simulink library "DEM_lib"  (Simulink 7.4)
settings: Solver=FixedStepDiscrete  StartTime=0.0  StopTime=Inf  FixedStep=0.001  RelTol=1e-3
undefined symbols (not defined in the file or in its folder): BCU_Drive_St, BCU_FastCharge_St, BCU_SlowCharge_St, COR_Fault_Bus, CTC_DefaultOffline_CtrCmd, CTC_DriveEmgyDcnct_CtrCmd, CTC_DriveOffline_CtrCmd, CTC_DriveOnline_CtrCmd, EHP_Fault_Bus, FCM_Fault_Bus, SCM_Fault_Bus
libraries: Defined_Functionality x82, simulink x2
(part 4 of 4)

== system DEM_lib/Diagnostic_Event_Management/Level_handle/DRIVE/FaultLevelConfirmed/LvlErr1 ==
  Err : Inport
  Bus Selector : BusSelector  OutputSignals=BPN_Fault_Bus.BPNd_cflt_CellVoltOver_warnRaw,BPN_Fault_Bus.BPNd_cflt_CellVoltUnder_warnRaw,BPN_Fault_Bus.BPNd_cflt_CellVoltDifOver_warnRaw,BPN_Fault_Bus.BPNd_cflt_PackVoltOver_warnRaw,BPN_Fault_Bus.BPNd_cflt_PackVoltUnder_warnRaw,BPN_Fault_Bus.BPNd_cflt_ChaCurOver_warnRaw,BPN_Fault_Bus.BPNd_cflt_DchCurOver_warnRaw,BPN_Fault_Bus.BPNd_cflt_PackSocUnder_warnRaw,BPN_Fault_Bus.BPNd_cflt_PackSocOver_warnRaw,BPN_Fault_Bus.BPNd_cflt_PulChaPowOver_warnRaw,BPN_Fault_Bus.BPNd_cflt_PulDchPowOver_warnRaw,BAL_Fault_Bus.BALd_cflt_BalSwthAnml_warnRaw,BTM_Fault_Bus.BTMd_cflt_MdlTempOver_warnRaw,BTM_Fault_Bus.BTMd_cflt_BMUMaxTempOver_warnRaw,BTM_Fault_Bus.BTMd_cflt_BCUMaxTempOver_warnRaw,BTM_Fault_Bus.BTMd_cflt_MdlTempUnder_warnRaw,BTM_Fault_Bus.BTMd_cflt_MdlTempDifOver_warnRaw,IPT_Fault_Bus.IPTd_cflt_CC2CnctSt_warnRaw,IPT_Fault_Bus.IPTd_cflt_CCCnctSt_warnRaw,IPT_Fault_Bus.IPTd_cflt_VMSCANMsg_faultRaw,IPT_Fault_Bus.IPTd_cflt_KL30Raw,IPT_Fault_Bus.IPTd_cflt_MSDVoltRaw,IPT_Fault_Bus.IPTd_cflt_PCBTempRaw,IPT_Fault_Bus.IPTd_cflt_PosCtrVoltRef1_backRaw,IPT_Fault_Bus.IPTd_cflt_PosCtrVoltRef1_frontRaw,IPT_Fault_Bus.IPTd_cflt_PosCtrVoltRef2_backRaw,IPT_Fault_Bus.IPTd_cflt_PosCtrVoltRef2_frontRaw,IPT_Fault_Bus.IPTd_cflt_ShuntCurRaw,IPT_Fault_Bus.IPTd_cflt_USampleRaw
  Constant : Constant  OutDataTypeMode=uint8  OutDataTypeStr=uint8
  Constant1 : Constant  Value=0  OutDataTypeMode=uint8  OutDataTypeStr=uint8
  Logical Operator : Logic  Operator=OR  Inputs=29  AllPortsSameDT=off  OutDataTypeMode=boolean  OutDataTypeStr=boolean
  Switch : Switch  Criteria=u2 ~= 0
  ErrLvl : Outport
  wires:
  Bus Selector/29 -> Logical Operator/29  "<IPTd_cflt_USampleRaw>"
  Bus Selector/28 -> Logical Operator/28  "<IPTd_cflt_ShuntCurRaw>"
  Bus Selector/27 -> Logical Operator/27  "<IPTd_cflt_PosCtrVoltRef2_frontRaw>"
  Bus Selector/26 -> Logical Operator/26  "<IPTd_cflt_PosCtrVoltRef2_backRaw>"
  Bus Selector/25 -> Logical Operator/25  "<IPTd_cflt_PosCtrVoltRef1_frontRaw>"
  Bus Selector/24 -> Logical Operator/24  "<IPTd_cflt_PosCtrVoltRef1_backRaw>"
  Bus Selector/23 -> Logical Operator/23  "<IPTd_cflt_PCBTempRaw>"
  Bus Selector/22 -> Logical Operator/22  "<IPTd_cflt_MSDVoltRaw>"
  Bus Selector/21 -> Logical Operator/21  "<IPTd_cflt_KL30Raw>"
  Bus Selector/20 -> Logical Operator/20  "<IPTd_cflt_VMSCANMsg_faultRaw>"
  Bus Selector/19 -> Logical Operator/19  "<IPTd_cflt_CCCnctSt_warnRaw>"
  Bus Selector/18 -> Logical Operator/18  "<IPTd_cflt_CC2CnctSt_warnRaw>"
  Bus Selector/17 -> Logical Operator/17  "<BTMd_cflt_MdlTempDifOver_warnRaw>"
  Bus Selector/16 -> Logical Operator/16  "<BTMd_cflt_MdlTempUnder_warnRaw>"
  Bus Selector/15 -> Logical Operator/15  "<BTMd_cflt_BCUMaxTempOver_warnRaw>"
  Bus Selector/14 -> Logical Operator/14  "<BTMd_cflt_BMUMaxTempOver_warnRaw>"
  Bus Selector/13 -> Logical Operator/13  "<BTMd_cflt_MdlTempOver_warnRaw>"
  Bus Selector/12 -> Logical Operator/12  "<BALd_cflt_BalSwthAnml_warnRaw>"
  Bus Selector/11 -> Logical Operator/11  "<BPNd_cflt_PulDchPowOver_warnRaw>"
  Bus Selector/10 -> Logical Operator/10  "<BPNd_cflt_PulChaPowOver_warnRaw>"
  Bus Selector/9 -> Logical Operator/9  "<BPNd_cflt_PackSocOver_warnRaw>"
  Bus Selector/8 -> Logical Operator/8  "<BPNd_cflt_PackSocUnder_warnRaw>"
  Bus Selector/7 -> Logical Operator/7  "<BPNd_cflt_DchCurOver_warnRaw>"
  Bus Selector/6 -> Logical Operator/6  "<BPNd_cflt_ChaCurOver_warnRaw>"
  Bus Selector/5 -> Logical Operator/5  "<BPNd_cflt_PackVoltUnder_warnRaw>"
  Bus Selector/4 -> Logical Operator/4  "<BPNd_cflt_PackVoltOver_warnRaw>"
  Bus Selector/3 -> Logical Operator/3  "<BPNd_cflt_CellVoltDifOver_warnRaw>"
  Bus Selector/2 -> Logical Operator/2  "<BPNd_cflt_CellVoltUnder_warnRaw>"
  Switch/1 -> ErrLvl/1
  Constant1/1 -> Switch/3
  Constant/1 -> Switch/1
  Logical Operator/1 -> Switch/2
  Err/1 -> Bus Selector/1
  Bus Selector/1 -> Logical Operator/1  "<BPNd_cflt_CellVoltOver_warnRaw>"

== system DEM_lib/Diagnostic_Event_Management/Level_handle/DRIVE/FaultLevelConfirmed/LvlErr2 ==
  Err : Inport
  Bus Selector : BusSelector  OutputSignals=BPN_Fault_Bus.BPNd_cflt_CellVoltOver_faultRaw,BPN_Fault_Bus.BPNd_cflt_CellVoltUnder_faultRaw,BPN_Fault_Bus.BPNd_cflt_CellVoltDifOver_faultRaw,BPN_Fault_Bus.BPNd_cflt_PackVoltOver_faultRaw,BPN_Fault_Bus.BPNd_cflt_PackVoltUnder_faultRaw,BPN_Fault_Bus.BPNd_cflt_ChaCurOver_faultRaw,BPN_Fault_Bus.BPNd_cflt_DchCurOver_faultRaw,BPN_Fault_Bus.BPNd_cflt_PackSocUnder_faultRaw,BPN_Fault_Bus.BPNd_cflt_PackSocOver_faultRaw,BPN_Fault_Bus.BPNd_cflt_PulChaPowOver_faultRaw,BPN_Fault_Bus.BPNd_cflt_PulDchPowOver_faultRaw,BPN_Fault_Bus.BPNd_cflt_PackInRes_fatalRaw,BPN_Fault_Bus.BPNd_cflt_HVPosCtrlR_faultRaw,BPN_Fault_Bus.BPNd_cflt_HVNegCtrlR_faultRaw,BPN_Fault_Bus.BPNd_cflt_HVAcq_warnRaw,EHP_Fault_Bus.EHPd_cflt_NegIso_warnRaw,EHP_Fault_Bus.EHPd_cflt_PosIso_warnRaw,COR_Fault_Bus.CORd_cflt_CellCDcse_faultRaw,COR_Fault_Bus.CORd_cflt_CellRDcse_faultRaw,COR_Fault_Bus.CORd_cflt_CellRIcse_faultRaw,BTM_Fault_Bus.BTMd_cflt_MdlTempOver_faultRaw,BTM_Fault_Bus.BTMd_cflt_MdlTempDifOver_faultRaw
  Constant : Constant  Value=2  OutDataTypeMode=uint8  OutDataTypeStr=uint8
  Constant1 : Constant  Value=0  OutDataTypeMode=uint8  OutDataTypeStr=uint8
  Logical Operator : Logic  Operator=OR  Inputs=22  AllPortsSameDT=off  OutDataTypeMode=boolean  OutDataTypeStr=boolean
  Switch : Switch  Criteria=u2 ~= 0
  ErrLvl : Outport
  wires:
  Bus Selector/22 -> Logical Operator/22  "<BTMd_cflt_MdlTempDifOver_faultRaw>"
  Bus Selector/21 -> Logical Operator/21  "<BTMd_cflt_MdlTempOver_faultRaw>"
  Bus Selector/20 -> Logical Operator/20  "<CORd_cflt_CellRIcse_faultRaw>"
  Bus Selector/19 -> Logical Operator/19  "<CORd_cflt_CellRDcse_faultRaw>"
  Bus Selector/18 -> Logical Operator/18  "<CORd_cflt_CellCDcse_faultRaw>"
  Bus Selector/17 -> Logical Operator/17  "<EHPd_cflt_PosIso_warnRaw>"
  Bus Selector/16 -> Logical Operator/16  "<EHPd_cflt_NegIso_warnRaw>"
  Bus Selector/15 -> Logical Operator/15  "<BPNd_cflt_HVAcq_warnRaw>"
  Bus Selector/14 -> Logical Operator/14  "<BPNd_cflt_HVNegCtrlR_faultRaw>"
  Bus Selector/13 -> Logical Operator/13  "<BPNd_cflt_HVPosCtrlR_faultRaw>"
  Bus Selector/12 -> Logical Operator/12  "<BPNd_cflt_PackInRes_fatalRaw>"
  Bus Selector/11 -> Logical Operator/11  "<BPNd_cflt_PulDchPowOver_faultRaw>"
  Bus Selector/10 -> Logical Operator/10  "<BPNd_cflt_PulChaPowOver_faultRaw>"
  Bus Selector/9 -> Logical Operator/9  "<BPNd_cflt_PackSocOver_faultRaw>"
  Bus Selector/8 -> Logical Operator/8  "<BPNd_cflt_PackSocUnder_faultRaw>"
  Bus Selector/7 -> Logical Operator/7  "<BPNd_cflt_DchCurOver_faultRaw>"
  Bus Selector/6 -> Logical Operator/6  "<BPNd_cflt_ChaCurOver_faultRaw>"
  Bus Selector/5 -> Logical Operator/5  "<BPNd_cflt_PackVoltUnder_faultRaw>"
  Bus Selector/4 -> Logical Operator/4  "<BPNd_cflt_PackVoltOver_faultRaw>"
  Bus Selector/3 -> Logical Operator/3  "<BPNd_cflt_CellVoltDifOver_faultRaw>"
  Bus Selector/2 -> Logical Operator/2  "<BPNd_cflt_CellVoltUnder_faultRaw>"
  Switch/1 -> ErrLvl/1
  Constant1/1 -> Switch/3
  Constant/1 -> Switch/1
  Bus Selector/1 -> Logical Operator/1  "<BPNd_cflt_CellVoltOver_faultRaw>"
  Err/1 -> Bus Selector/1
  Logical Operator/1 -> Switch/2

== system DEM_lib/Diagnostic_Event_Management/Level_handle/DRIVE/FaultLevelConfirmed/LvlErr3 ==
  Err : Inport
  Bus Selector : BusSelector  OutputSignals=BPN_Fault_Bus.BPNd_cflt_CellVoltOver_fatalRaw,BPN_Fault_Bus.BPNd_cflt_CellVoltUnder_fatalRaw,BPN_Fault_Bus.BPNd_cflt_PackVoltOver_fatalRaw,BPN_Fault_Bus.BPNd_cflt_PackVoltUnder_fatalRaw,BPN_Fault_Bus.BPNd_cflt_ChaCurOver_fatalRaw,BPN_Fault_Bus.BPNd_cflt_DchCurOver_fatalRaw,BPN_Fault_Bus.BPNd_cflt_PulChaPowOver_fatalRaw,BPN_Fault_Bus.BPNd_cflt_PulDchPowOver_fatalRaw,BPN_Fault_Bus.BPNd_cflt_PackVoltDrop_fatalRaw,CTC_Fault_Bus.CTCd_cflt_PosCtrStuckOpen_faultRaw,CTC_Fault_Bus.CTCd_cflt_PosCtrStuckCld_faultRaw,CTC_Fault_Bus.CTCd_cflt_NegCtrStuckOpen_faultRaw,CTC_Fault_Bus.CTCd_cflt_NegCtrStuckCld_faultRaw,CTC_Fault_Bus.CTCd_cflt_PrecTmOver_faultRaw,CTC_Fault_Bus.CTCd_cflt_HVCnctTmOver_faultRaw,CTC_Fault_Bus.CTCd_cflt_HVDcncWaitTmOver_faultRaw,CTC_Fault_Bus.CTCd_cflt_HVDcnctTmOver_faultRaw,CTC_Fault_Bus.CTCd_cflt_HVEmcyDcnctTmOver_faultRaw,CTC_Fault_Bus.CTCd_cflt_PrecCurOver_faultRaw,CTC_Fault_Bus.CTCd_cflt_HVCnctCurOver_faultRaw,EHP_Fault_Bus.EHPd_cflt_NegIso_faultRaw,EHP_Fault_Bus.EHPd_cflt_PosIso_faultRaw,EHP_Fault_Bus.EHPd_cflt_HVILSt_faultRaw,BTM_Fault_Bus.BTMd_cflt_MdlTempOver_fatalRaw,BSC_Fault_Bus.BSCd_cflt_BCUFaultRaw,MCC_Fault_Bus.MCCd_cflt_BMUInit_faultRaw
  Constant : Constant  Value=3  OutDataTypeMode=uint8  OutDataTypeStr=uint8
  Constant1 : Constant  Value=0  OutDataTypeMode=uint8  OutDataTypeStr=uint8
  Logical Operator1 : Logic  Operator=OR  Inputs=26  AllPortsSameDT=off  OutDataTypeMode=boolean  OutDataTypeStr=boolean
  Switch : Switch  Criteria=u2 ~= 0
  ErrLvl : Outport
  wires:
  Bus Selector/26 -> Logical Operator1/26  "<MCCd_cflt_BMUInit_faultRaw>"
  Bus Selector/25 -> Logical Operator1/25  "<BSCd_cflt_BCUFaultRaw>"
  Bus Selector/24 -> Logical Operator1/24  "<BTMd_cflt_MdlTempOver_fatalRaw>"
  Bus Selector/23 -> Logical Operator1/23  "<EHPd_cflt_HVILSt_faultRaw>"
  Bus Selector/22 -> Logical Operator1/22  "<EHPd_cflt_PosIso_faultRaw>"
  Bus Selector/21 -> Logical Operator1/21  "<EHPd_cflt_NegIso_faultRaw>"
  Bus Selector/20 -> Logical Operator1/20  "<CTCd_cflt_HVCnctCurOver_faultRaw>"
  Bus Selector/19 -> Logical Operator1/19  "<CTCd_cflt_PrecCurOver_faultRaw>"
  Bus Selector/18 -> Logical Operator1/18  "<CTCd_cflt_HVEmcyDcnctTmOver_faultRaw>"
  Bus Selector/17 -> Logical Operator1/17  "<CTCd_cflt_HVDcnctTmOver_faultRaw>"
  Bus Selector/16 -> Logical Operator1/16  "<CTCd_cflt_HVDcncWaitTmOver_faultRaw>"
  Bus Selector/15 -> Logical Operator1/15  "<CTCd_cflt_HVCnctTmOver_faultRaw>"
  Bus Selector/14 -> Logical Operator1/14  "<CTCd_cflt_PrecTmOver_faultRaw>"
  Bus Selector/13 -> Logical Operator1/13  "<CTCd_cflt_NegCtrStuckCld_faultRaw>"
  Bus Selector/12 -> Logical Operator1/12  "<CTCd_cflt_NegCtrStuckOpen_faultRaw>"
  Bus Selector/11 -> Logical Operator1/11  "<CTCd_cflt_PosCtrStuckCld_faultRaw>"
  Bus Selector/10 -> Logical Operator1/10  "<CTCd_cflt_PosCtrStuckOpen_faultRaw>"
  Bus Selector/9 -> Logical Operator1/9  "<BPNd_cflt_PackVoltDrop_fatalRaw>"
  Bus Selector/8 -> Logical Operator1/8  "<BPNd_cflt_PulDchPowOver_fatalRaw>"
  Bus Selector/7 -> Logical Operator1/7  "<BPNd_cflt_PulChaPowOver_fatalRaw>"
  Bus Selector/6 -> Logical Operator1/6  "<BPNd_cflt_DchCurOver_fatalRaw>"
  Bus Selector/5 -> Logical Operator1/5  "<BPNd_cflt_ChaCurOver_fatalRaw>"
  Bus Selector/4 -> Logical Operator1/4  "<BPNd_cflt_PackVoltUnder_fatalRaw>"
  Bus Selector/3 -> Logical Operator1/3  "<BPNd_cflt_PackVoltOver_fatalRaw>"
  Bus Selector/2 -> Logical Operator1/2  "<BPNd_cflt_CellVoltUnder_fatalRaw>"
  Switch/1 -> ErrLvl/1
  Constant1/1 -> Switch/3
  Constant/1 -> Switch/1
  Logical Operator1/1 -> Switch/2
  Err/1 -> Bus Selector/1
  Bus Selector/1 -> Logical Operator1/1  "<BPNd_cflt_CellVoltOver_fatalRaw>"

== system DEM_lib/Diagnostic_Event_Management/Level_handle/DRIVE/handle/DriveCtrCmdRaw ==
  BSCd_enum_BCUSt : Inport
  IPTd_flg_VehHVCnctCmd : Inport  Port=2
  Compare To Constant4 : simulink/Logic and Bit Operations/Compare To Constant  SystemSampleTime=-1  relop===  const=BCU_Drive_St  LogicOutDataTypeMode=uint8
  Compare To Constant5 : simulink/Logic and Bit Operations/Compare To Constant  SystemSampleTime=-1  relop===  const=1  LogicOutDataTypeMode=uint8
  Constant1 : Constant  Value=CTC_DriveOffline_CtrCmd  OutDataTypeMode=uint8  OutDataTypeStr=uint8
  Constant2 : Constant  Value=CTC_DriveOnline_CtrCmd  OutDataTypeMode=uint8  OutDataTypeStr=uint8
  Logical Operator3 : Logic  AllPortsSameDT=off  OutDataTypeMode=boolean  OutDataTypeStr=boolean
  Switch2 : Switch  Criteria=u2 ~= 0  OutDataTypeMode=single  OutDataTypeStr=single
  DEMd_enum_DrvCtrCmdRaw : Outport  OutDataType=fixdt(1, 16)  OutScaling=2^0
  wires:
  Switch2/1 -> DEMd_enum_DrvCtrCmdRaw/1  "DEMd_enum_DrvCtrCmdRaw"
  IPTd_flg_VehHVCnctCmd/1 -> Compare To Constant5/1
  Compare To Constant4/1 -> Logical Operator3/1
  Compare To Constant5/1 -> Logical Operator3/2
  Constant2/1 -> Switch2/1
  Logical Operator3/1 -> Switch2/2
  BSCd_enum_BCUSt/1 -> Compare To Constant4/1
  Constant1/1 -> Switch2/3

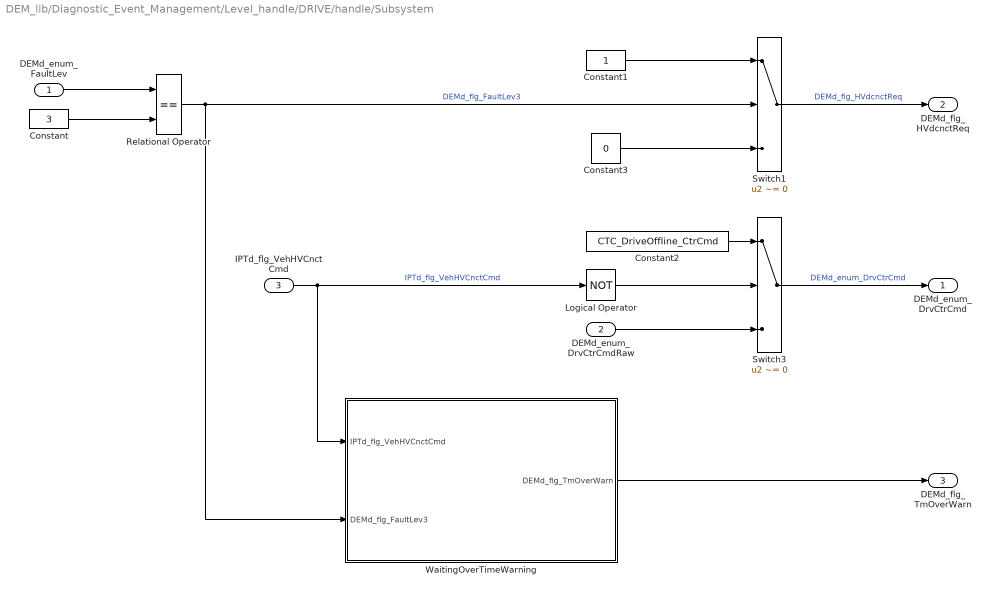
== system DEM_lib/Diagnostic_Event_Management/Level_handle/DRIVE/handle/Subsystem ==
  DEMd_enum_FaultLev : Inport
  DEMd_enum_DrvCtrCmdRaw : Inport  Port=2
  IPTd_flg_VehHVCnctCmd : Inport  Port=3
  Constant : Constant  Value=3  OutDataType=fixdt(1, 16)  OutScaling=2^0
  Constant1 : Constant  OutDataTypeMode=boolean  OutDataType=fixdt(1, 16)  OutScaling=2^0  OutDataTypeStr=boolean
  Constant2 : Constant  Value=CTC_DriveOffline_CtrCmd  OutDataTypeMode=uint8  OutDataTypeStr=uint8
  Constant3 : Constant  Value=0  OutDataTypeMode=boolean  OutDataType=fixdt(1, 16)  OutScaling=2^0  OutDataTypeStr=boolean
  Logical Operator : Logic  Operator=NOT  Inputs=1  AllPortsSameDT=off  OutDataTypeMode=boolean  LogicDataType=fixdt(0, 8)  OutDataTypeStr=boolean
  Relational Operator : RelationalOperator  Operator===  LogicOutDataTypeMode=boolean  LogicDataType=fixdt(0, 8)  OutDataTypeStr=boolean
  Switch1 : Switch  Criteria=u2 ~= 0
  Switch3 : Switch  Criteria=u2 ~= 0
  WaitingOverTimeWarning : Stateflow chart  Description=|  TreatAsAtomicUnit=on
      | $Author:Yan LiJuan$
      | $Date:2015/03/26$  
      | $Revision:1.0$
  DEMd_enum_DrvCtrCmd : Outport
  DEMd_flg_HVdcnctReq : Outport  Port=2  OutDataType=fixdt(1, 16)  OutScaling=2^0
  DEMd_flg_TmOverWarn : Outport  Port=3
  wires:
  Logical Operator/1 -> Switch3/2
  Constant3/1 -> Switch1/3
  Relational Operator/1 -> Switch1/2, WaitingOverTimeWarning/2(DEMd_flg_FaultLev3)  "DEMd_flg_FaultLev3"
  DEMd_enum_FaultLev/1 -> Relational Operator/1
  WaitingOverTimeWarning/1(DEMd_flg_TmOverWarn) -> DEMd_flg_TmOverWarn/1
  Switch1/1 -> DEMd_flg_HVdcnctReq/1  "DEMd_flg_HVdcnctReq"
  Constant1/1 -> Switch1/1
  Constant/1 -> Relational Operator/2
  IPTd_flg_VehHVCnctCmd/1 -> Logical Operator/1, WaitingOverTimeWarning/1(IPTd_flg_VehHVCnctCmd)  "IPTd_flg_VehHVCnctCmd"
  DEMd_enum_DrvCtrCmdRaw/1 -> Switch3/3
  Switch3/1 -> DEMd_enum_DrvCtrCmd/1  "DEMd_enum_DrvCtrCmd"
  Constant2/1 -> Switch3/1

== system DEM_lib/Diagnostic_Event_Management/Level_handle/DRIVE/handle/serious 1 ==
  DEMd_cflt_fault : Inport
  DEMd_enum_FaultLev : Inport  Port=2
  DEMd_enum_DrvCtrCmd : Inport  Port=3
  Bus Selector : BusSelector  OutputSignals=IPT_Fault_Bus.IPTd_cflt_VMSCANMsg_faultRaw
  Constant : Constant  Value=3  OutDataType=fixdt(1, 16)  OutScaling=2^0
  Constant3 : Constant  Value=CTC_DriveEmgyDcnct_CtrCmd  OutDataTypeMode=uint8  OutDataTypeStr=uint8  LockScale=on
  Logical Operator2 : Logic  AllPortsSameDT=off  OutDataTypeMode=boolean  OutDataTypeStr=boolean
  Relational Operator : RelationalOperator  Operator===  LogicOutDataTypeMode=boolean  LogicDataType=fixdt(0, 8)  OutDataTypeStr=boolean
  Switch3 : Switch  Criteria=u2 ~= 0
  DEMd_enum_CtrCmdRaw : Outport
  wires:
  Relational Operator/1 -> Logical Operator2/1
  Constant3/1 -> Switch3/1
  Logical Operator2/1 -> Switch3/2
  Switch3/1 -> DEMd_enum_CtrCmdRaw/1  "DEMd_enum_CtrCmdRaw"
  DEMd_cflt_fault/1 -> Bus Selector/1
  DEMd_enum_DrvCtrCmd/1 -> Switch3/3
  DEMd_enum_FaultLev/1 -> Relational Operator/1
  Constant/1 -> Relational Operator/2
  Bus Selector/1 -> Logical Operator2/2  "<IPTd_cflt_VMSCANMsg_faultRaw>"

== stateflow chart Diagnostic_Event_Management/Level_handle/DRIVE/handle/Subsystem/WaitingOverTimeWarning ==
  settings: description=|
      | $Author:Yan LiJuan$
      | $Date:2015/03/26$
      | $Revision:1.0$
  state Off
    DEMd_flg_TmOverWarn=0;
  state Wait
    (default) -> (junction 6) : {Timer_On=0;}
    Wait -> (junction 6) [order 1]
    (junction 6) -> (junction 7) : {Timer_On++;}
  state On
    DEMd_flg_TmOverWarn=1;
  (default) -> Off
  Off -> Wait : [(DEMd_flg_FaultLev3==1)&&...
      | (IPTd_flg_VehHVCnctCmd==1)]
  Wait -> On [order 2] : [Timer_On>=DEMc_tm_TmOverWarn]
  On -> Off : [IPTd_flg_VehHVCnctCmd==0]
  Wait -> Off [order 1] : [IPTd_flg_VehHVCnctCmd==0]
  data: Timer_On local double; IPTd_flg_VehHVCnctCmd input boolean; DEMd_flg_FaultLev3 input boolean; DEMc_tm_TmOverWarn parameter uint16; DEMd_flg_TmOverWarn output boolean
